simulink model "forloopsf"  (Simulink 7.1)
settings: Solver=FixedStepDiscrete  StartTime=0.0  StopTime=20  FixedStep=.01  RelTol=1e-3
settings Model: Creator=ajayaram  LastModifiedBy=ajayaram
settings OptimizationCC: InlineParams=on  OptimizeModelRefInitCode=on  LifeSpan=1
settings DebuggingCC: SaveWithParameterizedLinksMsg=none
settings RTWCC: SystemTargetFile=ert.tlc  GenCodeOnly=on  GenerateMakefile=off  TemplateMakefile=ert_default_tmf  Description=Real-Time Workshop Embedded Coder (no auto configuration)  GenerateReport=on  ProcessScript=ert_make_rtw_hook  IncludeHyperlinkInReport=on  LaunchReport=on
settings CodeAppCC: GenerateComments=off  IgnoreCustomStorageClasses=off  SimulinkBlockComments=off
settings ERTTargetCC: TargetFcnLib=ansi_tfl_tmw.mat  InlinedParameterPlacement=NonHierarchical  ERTCustomFileTemplate=example_file_process.tlc

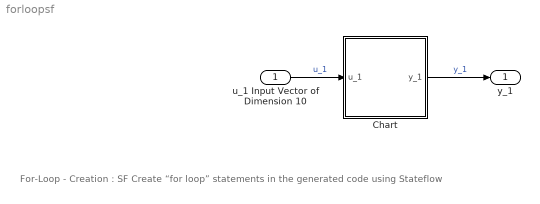
== system forloopsf ==
  note: For-Loop - Creation : SF
      | Create “for loop” statements in the
      | generated code using Stateflow
  u_1 Input Vector of Dimension 10 : Inport  PortDimensions=10  OutDataType=sfix(16)  OutScaling=2^0
  Chart : Stateflow chart
  y_1 : Outport  OutDataType=sfix(16)  OutScaling=2^0
  wires:
  u_1 Input Vector of Dimension 10/1 -> Chart/1(u_1)  "u_1"
  Chart/1(y_1) -> y_1/1  "y_1"

== stateflow chart Chart ==
  (junction 6) -> (junction 4) : {
      | inx++;
      | }
  (default) -> (junction 4) : {
      | inx =0;
      | }
  (junction 4) -> (junction 3) [order 2]
  (junction 4) -> (junction 5) [order 1] : [inx<10]
  (junction 5) -> (junction 6) : {
      | y_1 = u_1[inx] + y_1 ;
      | }
  data: u_1 input double; y_1 output double =0; inx local double
